simulink model "ask2"  (R2020a)
settings: Solver=VariableStepAuto  StartTime=0.0  StopTime=10.0  RelTol=1e-3
undefined symbols (not defined in the file): fdesignblkfcn, gcbh
libraries: commutil2 x3, commchan3 x2, commdigbbndam3 x2, commsink2 x1, dspfdesign x1
settings Model: Creator=王豪666  LastModifiedBy=王豪666

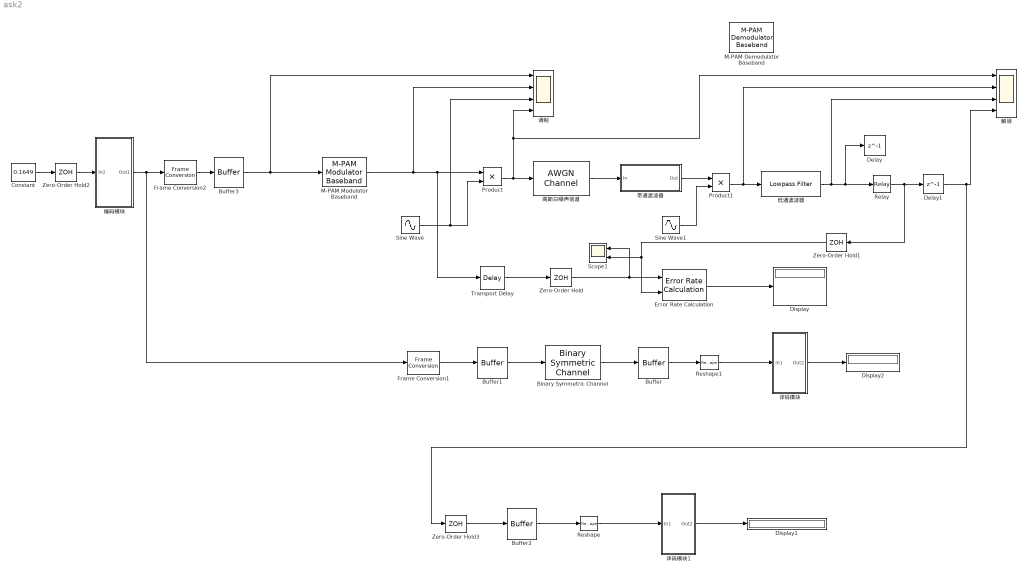
== system ask2 ==
  Binary Symmetric Channel : commchan3/Binary Symmetric Channel  ErrorProbability=0  ErrorVectorOutputPort=off  OutputDataType=double  OutputDataTypeSL=double  Seed=71  SimulateUsing=Code generation
      settings: SourceProductBaseCode=CM
  Buffer : Buffer  N=8  OutputFrames=off
  Buffer1 : Buffer  N=1  OutputFrames=off
  Buffer2 : Buffer  N=8  OutputFrames=off
  Buffer3 : Buffer  N=1  OutputFrames=off
  Constant : Constant  Value=0.1649
  Delay : Delay  DelayLength=1
  Delay1 : Delay  DelayLength=1
  Display : Display
  Display1 : Display
  Display2 : Display
  Error Rate Calculation : commsink2/Error Rate Calculation  N=0  st_delay=0  cp_mode=Entire frame  subframe=[]  PMode=Port  WsName=ErrorVec  RsMode2=off  stop=off  numErr=100  maxBits=1e6
  Frame Conversion1 : FrameConversion
  Frame Conversion2 : FrameConversion
  M-PAM Demodulator Baseband : commdigbbndam3/M-PAM Demodulator Baseband  M=4  OutType=Integer  Dec=Gray  PowType=Min. distance between symbols  MinDist=2  AvgPow=1  PeakPow=1  outDtype1=Inherit via internal rule  outDtype2=Inherit via internal rule  denormFactorWordLen=16  denormFactorDataTypeStr=Inherit: Same word length as input  denormFactorLastDataTypeStr=Inherit: Same word length as input  prodOutWordLen=16  prodOutRoundingMode=Floor  prodOutOverflowMode=Wrap  prodOutOvFlMode=off  prodOutOvFlModeLastStrValue=off  sumWordLen=16
      settings: SourceProductBaseCode=CM
  M-PAM Modulator Baseband : commdigbbndam3/M-PAM Modulator Baseband  M=2  InType=Integer  Enc=Gray  PowType=Min. distance between symbols  MinDist=2  AvgPow=1  PeakPow=1  outDtype=double  outWordLen=16  outUDDataType=sfix(16)  outFracLenMode=Best precision  outFracLen=15  outDataTypeStr=double  outLastDataTypeStr=double
      settings: SourceProductBaseCode=CM
  Product : Product
  Product1 : Product
  Relay : Relay
  Reshape : Reshape
  Reshape1 : Reshape
  Scope1 : Scope  NumInputPorts=2
  Sine Wave : Sin  Frequency=4*2*pi  SampleTime=0.01
  Sine Wave1 : Sin  Frequency=4*2*pi  SampleTime=0.01
  Transport Delay : TransportDelay  DelayTime=2.68
  Zero-Order Hold : ZeroOrderHold  SampleTime=-1
  Zero-Order Hold1 : ZeroOrderHold  SampleTime=-1
  Zero-Order Hold2 : ZeroOrderHold  SampleTime=9
  Zero-Order Hold3 : ZeroOrderHold
  低通滤波器 : dspfdesign/Lowpass Filter  FilterType=FIR  DesignForMinimumOrder=on  FilterOrder=50  PassbandFrequency=1  StopbandFrequency=100  PassbandRipple=1  StopbandAttenuation=60  InheritSampleRate=off  SampleRate=6000  SimulateUsing=Interpreted execution  roundingMode=Floor  coeffsDataTypeStr=fixdt(1,16)
  带通滤波器 : Subsystem  DialogController=fdesignblkfcn  InitFcn=fdesignblkfcn(gcbh, {'InitFcn'});  mask(Bandpass Filter){}
      mask help: Design a bandpass filter
      settings: CopyFcn=fdesignblkfcn(gcbh, {'CopyFcn'});
      mask Help: helpview(mapfilelocation('dsp'), 'dspbandpassfilter');
      mask Display: disp('Bandpass');
  编码模块 : Subsystem
  解调 : Scope  NumInputPorts=4
  译码模块 : Subsystem
  译码模块1 : Subsystem
  调制 : Scope  NumInputPorts=4
  高斯白噪声信道 : commchan3/AWGN Channel  InputProcessing=Columns as channels (frame based)  seed=67  noiseMode="Signal to noise ratio  (Eb/No)"  EbNodB=35  EsNodB=10  SNRdB=10  bitsPerSym=1  Ps=1  Tsym=1  variance=1
  wires:
  Product/1 -> 解调/1, 调制/4, 高斯白噪声信道/1
  高斯白噪声信道/1 -> 带通滤波器/1(In)
  带通滤波器/1(Out) -> Product1/1
  Product1/1 -> 解调/2, 低通滤波器/1
  低通滤波器/1 -> 解调/3, Delay/1, Relay/1
  Relay/1 -> Zero-Order Hold1/1, Delay1/1
  Zero-Order Hold2/1 -> 编码模块/1(In2)
  Transport Delay/1 -> Zero-Order Hold/1
  Sine Wave1/1 -> Product1/2
  Zero-Order Hold1/1 -> Scope1/2, Error Rate Calculation/2
  Error Rate Calculation/1 -> Display/1
  Zero-Order Hold/1 -> Scope1/1, Error Rate Calculation/1
  Constant/1 -> Zero-Order Hold2/1
  Zero-Order Hold3/1 -> Buffer2/1
  Buffer2/1 -> Reshape/1
  Reshape/1 -> 译码模块1/1(In1)
  译码模块1/1(Out2) -> Display1/1
  Frame Conversion1/1 -> Buffer1/1
  Buffer1/1 -> Binary Symmetric Channel/1
  Binary Symmetric Channel/1 -> Buffer/1
  Buffer/1 -> Reshape1/1
  Reshape1/1 -> 译码模块/1(In1)
  译码模块/1(Out2) -> Display2/1
  Frame Conversion2/1 -> Buffer3/1
  编码模块/1(Out1) -> Frame Conversion2/1, Frame Conversion1/1
  Sine Wave/1 -> 调制/3, Product/2
  Buffer3/1 -> 调制/1, M-PAM Modulator Baseband/1
  M-PAM Modulator Baseband/1 -> 调制/2, Transport Delay/1, Product/1
  Delay1/1 -> Zero-Order Hold3/1, 解调/4

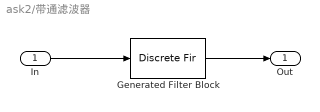
== system ask2/带通滤波器 ==
  In : Inport
  Generated Filter Block : DiscreteFir  Tag=BlockMethodSubSystem  Coefficients=[0.000542653428276014841 -0.000203430595301854356 -0.00015082179928837603 -9.50845869135781216e-05 -3.45888711570517711e-05 3.20867019503190149e-05 0.000105351948236212913 0.000183604020004364023 0.000263095866697428426 0.000337607345421654789 0.000399143453211069283 0.000438308061388886479 0.000445663411873770663 0.000412549440751391069 0.000332743561617878812 0.000203221396324684833 2.55857826470748135e-05 -0.000193849247887811684 -0.000442949242881924686 -0.000706373686619458929 -0.000961052506708613219 -0.00118758887784600211 -0.00135937740359867178 -0.00145442196424048304 -0.00145522834677436859 -0.00134868271753454255 -0.0011290387434029197 -0.000799963105418745888 -0.000375084783267701596 0.000122665157915531826 0.00066239206682439729 0.00120697786808646049 0.00171562944890786659 0.00214686024346833967 0.00246216384643116893 0.0026294097596439108 0.00262626431217770871 0.00244231867457264228 0.00208136976846043376 0.00156035958162383534 0.000911043134928900137 0.000174896602252948481 -0.00059716337976223441 -0.00134978515535131563 -0.00202822960528270101 -0.00258191881167479237 -0.00296897808325484935 -0.00316034745779216137 -0.00314236351272836369 -0.00291789073634860126 -0.00250617163201750188 -0.00194147393166935254 -0.00127013182651115756 -0.00054647157352106482 0.000172219928363430658 0.000830697186256610645 0.00138085879800946992 0.00178564942425432898 0.00202300604211833523 0.00208667445917749741 0.00198779076422466415 0.00175220997315741426 0.00141815240596848582 0.00103218200250870221 0.00064355951391778098 0.000299311654266077101 3.92334027874458209e-05 -0.000108763068050162404 -0.000131790405299620048 -3.34404316215393231e-05 0.000166483161036354321 0.000433823278382122215 0.000723768327886330025 0.000985795510863390467 0.00116951411346465127 0.00123040023454243494 0.00113545594179133985 0.000867302211144848918 0.000427736204569782892 -0.000161957345029091785 -0.000861416529448356624 -0.00161471042757097851 -0.0023553048793943294 -0.00301191402626231489 -0.00351587705112784126 -0.00380819405377857793 -0.00384574221978978628 -0.00360648511098966102 -0.00309260257890437568 -0.00233122867470514708 -0.00137272955397655131 -0.000286812789747891328 0.000843544310873414359 0.00192961161817751105 0.00288529327744900446 0.00363516753450304894 0.00412200914755440385 0.00431208435495056015 0.00419897042258551238 0.00380379476525621093 0.00317333457347117581 0.00237530734352075709 0.00149120654515740459 0.000608172796636916404 -0.000190227714802306707 -0.00083293145745540957 -0.00126875799385687367 -0.00147197364834850326 -0.0014451321745417875 -0.0012188121899442694 -0.000848199449962231755 -0.000406998442703239297 2.09932440479607347e-05 0.000351653443252821169 0.000510773584148355945 0.000443270113983067345 0.000121004100410941195 -0.000452579176527548701 -0.00124055716110878667 -0.00217476365112841824 -0.00316146473083048045 -0.00408992808672413791 -0.00484373155827680021 -0.00531296484451874475 -0.00540651315588196527 -0.00506323609791767271 -0.00426032142165878695 -0.00301825148196107349 -0.00140162086598064018 0.000484542809955304564 0.00250282614168851779 0.00449501116835118297 0.00629631697262520058 0.00775084852780537001 0.00872691706023674164 0.00913026503555437394 0.00891442647787287282 0.00808632940108428011 0.00670710627816910147 0.00488743804045808222 0.00277768716133301556 0.000554189775296216294 -0.00159767343106772034 -0.00350160206325748988 -0.00500782122437009019 -0.00600843226940829533 -0.00644855624715500852 -0.0063322128376336103 -0.0057222190798380014 -0.0047338323554613022 -0.00352253306871086426 -0.00226718677991902999 -0.00115009533593642913 -0.000336010560143632734 4.79191611979026821e-05 -7.13344339468600453e-05 -0.000701073572061241342 -0.00177816652101939481 -0.00317179321818048324 -0.00469368036336244299 -0.00611559427354856078 -0.00719209871043956055 -0.00768691608297853574 -0.00740041119063926996 -0.00619506294235536333 -0.0040166736098995303 -0.000908606804279565861 ...(+5379 chars)]  InputProcessing=Columns as channels (frame based)
  Out : Outport  VectorParamsAs1DForOutWhenUnconnected=off
  wires:
  In/1 -> Generated Filter Block/1
  Generated Filter Block/1 -> Out/1

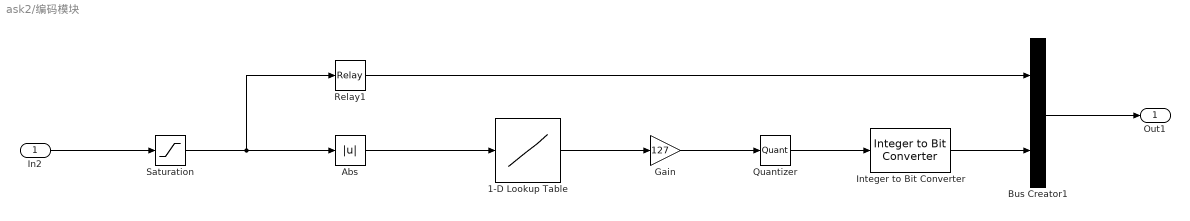
== system ask2/编码模块 ==
  In2 : Inport
  1-D Lookup Table : Lookup_n-D  NumberOfTableDimensions=1  BreakpointsForDimension1=[-1,-1/2,-1/4,-1/8,-1/16,-1/32,-1/64,-1/128,0,1/128,1/64,1/32,1/16,1/8,1/4,1/2,1]  Table=[-1,-7/8,-6/8,-5/8,-4/8,-3/8,-2/8,-1/8,0,1/8,2/8,3/8,4/8,5/8,6/8,7/8,1]  InternalRulePriority=Speed  RndMeth=Simplest  InputSameDT=on
  Abs : Abs
  Bus Creator1 : BusCreator  Inputs=2
  Gain : Gain  Gain=127
  Integer to Bit Converter : commutil2/Integer to Bit Converter  nbits=7  signedInputValues=Unsigned  bitOrder=MSB first  outDtype=Inherit via internal rule
  Quantizer : Quantizer  QuantizationInterval=1
  Relay1 : Relay
  Saturation : Saturate  UpperLimit=1  LowerLimit=-1
  Out1 : Outport
  wires:
  Integer to Bit Converter/1 -> Bus Creator1/2
  Bus Creator1/1 -> Out1/1
  Gain/1 -> Quantizer/1
  In2/1 -> Saturation/1
  1-D Lookup Table/1 -> Gain/1
  Relay1/1 -> Bus Creator1/1
  Quantizer/1 -> Integer to Bit Converter/1
  Abs/1 -> 1-D Lookup Table/1
  Saturation/1 -> Relay1/1, Abs/1

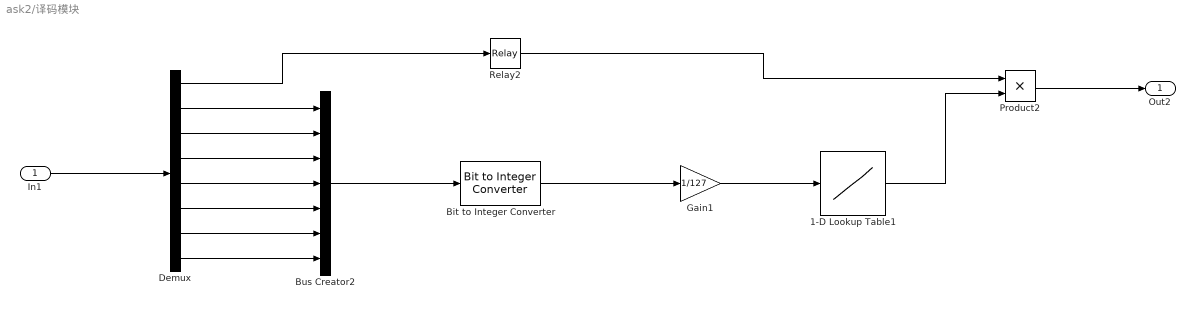
== system ask2/译码模块 ==
  In1 : Inport
  1-D Lookup Table1 : Lookup_n-D  NumberOfTableDimensions=1  BreakpointsForDimension1=[-1,-7/8,-6/8,-5/8,-4/8,-3/8,-2/8,-1/8,0,1/8,2/8,3/8,4/8,5/8,6/8,7/8,1]  Table=[-1,-1/2,-1/4,-1/8,-1/16,-1/32,-1/64,-1/128,0,1/128,1/64,1/32,1/16,1/8,1/4,1/2,1]  InternalRulePriority=Speed  RndMeth=Simplest  InputSameDT=on
  Bit to Integer Converter : commutil2/Bit to Integer Converter  nbits=7  bitOrder=MSB first  signedOutputValues=Unsigned  outDtype=Inherit via internal rule  outDtypeSigned=Inherit via internal rule
  Bus Creator2 : BusCreator  Inputs=7
  Demux : Demux  Outputs=8
  Gain1 : Gain  Gain=1/127
  Product2 : Product
  Relay2 : Relay
  Out2 : Outport
  wires:
  Demux/7 -> Bus Creator2/6
  Bit to Integer Converter/1 -> Gain1/1
  Bus Creator2/1 -> Bit to Integer Converter/1
  Product2/1 -> Out2/1
  Demux/5 -> Bus Creator2/4
  Demux/6 -> Bus Creator2/5
  Demux/3 -> Bus Creator2/2
  Demux/4 -> Bus Creator2/3
  1-D Lookup Table1/1 -> Product2/2
  Demux/1 -> Relay2/1
  Gain1/1 -> 1-D Lookup Table1/1
  Demux/8 -> Bus Creator2/7
  Demux/2 -> Bus Creator2/1
  Relay2/1 -> Product2/1
  In1/1 -> Demux/1

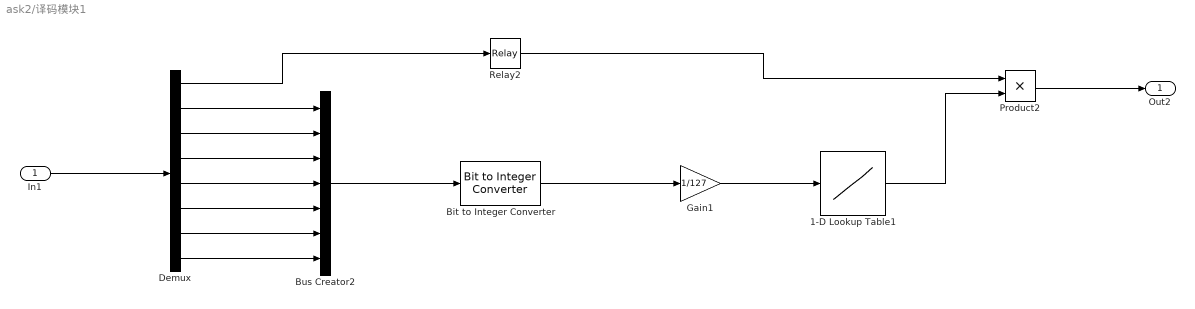
== system ask2/译码模块1 ==
  In1 : Inport
  1-D Lookup Table1 : Lookup_n-D  NumberOfTableDimensions=1  BreakpointsForDimension1=[-1,-7/8,-6/8,-5/8,-4/8,-3/8,-2/8,-1/8,0,1/8,2/8,3/8,4/8,5/8,6/8,7/8,1]  Table=[-1,-1/2,-1/4,-1/8,-1/16,-1/32,-1/64,-1/128,0,1/128,1/64,1/32,1/16,1/8,1/4,1/2,1]  InternalRulePriority=Speed  RndMeth=Simplest  InputSameDT=on
  Bit to Integer Converter : commutil2/Bit to Integer Converter  nbits=7  bitOrder=MSB first  signedOutputValues=Unsigned  outDtype=Inherit via internal rule  outDtypeSigned=Inherit via internal rule
  Bus Creator2 : BusCreator  Inputs=7
  Demux : Demux  Outputs=8
  Gain1 : Gain  Gain=1/127
  Product2 : Product
  Relay2 : Relay
  Out2 : Outport
  wires:
  Demux/7 -> Bus Creator2/6
  Bit to Integer Converter/1 -> Gain1/1
  Bus Creator2/1 -> Bit to Integer Converter/1
  Product2/1 -> Out2/1
  Demux/5 -> Bus Creator2/4
  Demux/6 -> Bus Creator2/5
  Demux/3 -> Bus Creator2/2
  Demux/4 -> Bus Creator2/3
  1-D Lookup Table1/1 -> Product2/2
  Demux/1 -> Relay2/1
  Gain1/1 -> 1-D Lookup Table1/1
  Demux/8 -> Bus Creator2/7
  Demux/2 -> Bus Creator2/1
  Relay2/1 -> Product2/1
  In1/1 -> Demux/1
